simulink model "ultimate_lqr"  (R2023a)
settings: Solver=VariableStepAuto  StartTime=0.0  StopTime=10.0  RelTol=1e-3
values from neighbouring files (symbols this model uses):
  Ard = [Ar(1,1) Ar(1,3:end) ... (first row only)    [Modelo_mono.m]    (also in workspace.mat = [0 0 -31.2551437046 31.2551437046 0 0 0 0 0 0 -92.3888975157)
  Brd = [Br(1,:) ... (first row only)    [Modelo_mono.m]    (also in workspace.mat = [0  0; 0  0; 50297.8358889  0; -78.116759971  0; 0  238.3657)
  Crd = [1 0 0 0 0 0 0 1 0 0 0 0 ... (36 elements, 6x6)]    [workspace.mat]
  K = lqr(Ard,Brd,Qc,Rc)    [Modelo_mono.m]    (also in cascatinha_v3.m = [tprK,0; workspace.mat = [-891.058429104  -1.00065730536e-12  -0.217264538579  -159.5)
  v_ic = [0;0;0;0]    [Modelo_mono.m]    (also in workspace.mat = [0 0 0 0])
  x_ic = [0;5*pi/180;0;-5*pi/180]    [Modelo_mono.m]    (also in workspace.mat = [0 0.0872664625997 0 -0.0872664625997])
libraries: simulink_extras x1
settings Model: Creator=pinki  LastModifiedBy=pinki

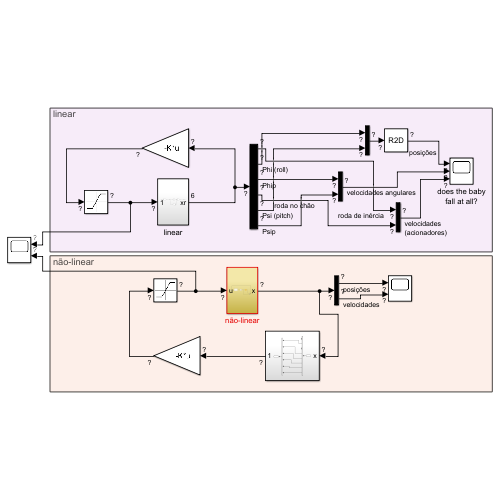
[thumbnail: Simulink's stored preview of the top-level diagram]
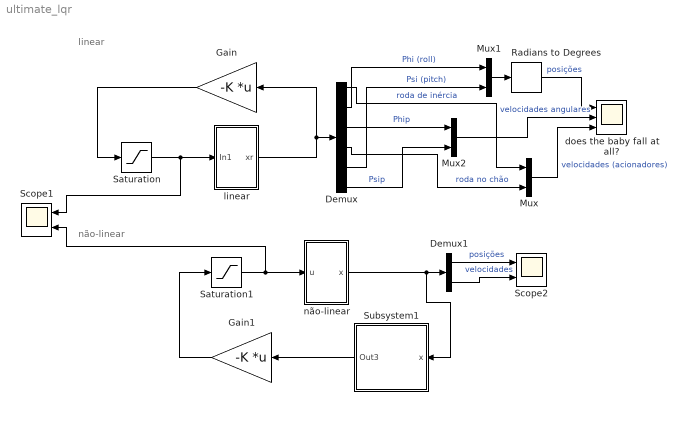
== system ultimate_lqr ==
  note: não-linear
  note: linear
  Demux : Demux  Outputs=6
  Demux1 : Demux  Outputs=2
  Gain : Gain  Gain=-K  Multiplication=Matrix(K*u)
  Gain1 : Gain  Gain=-K  Multiplication=Matrix(K*u)
  Mux : Mux  Inputs=2
  Mux1 : Mux  Inputs=2
  Mux2 : Mux  Inputs=2
  Radians to Degrees : simulink_extras/Transformations/Radians to Degrees
  Saturation : Saturate  UpperLimit=1  LowerLimit=-1
  Saturation1 : Saturate  UpperLimit=1  LowerLimit=-1
  Scope1 : Scope  NumInputPorts=2
  Scope2 : Scope  NumInputPorts=2
  Subsystem1 : Subsystem
  does the baby fall at all? : Scope  NumInputPorts=3
  linear : Subsystem
  não-linear : Subsystem
  wires:
  linear/1(xr) -> Gain/1, Demux/1
  Saturation/1 -> Scope1/1, linear/1(In1)
  Demux1/2 -> Scope2/2  "velocidades"
  Demux1/1 -> Scope2/1  "posições"
  não-linear/1(x) -> Subsystem1/1(x), Demux1/1
  Gain/1 -> Saturation/1
  Subsystem1/1(Out3) -> Gain1/1
  Gain1/1 -> Saturation1/1
  Saturation1/1 -> não-linear/1(u), Scope1/2
  Demux/1 -> Mux/1  "roda de inércia"
  Mux2/1 -> does the baby fall at all?/2  "velocidades angulares"
  Mux1/1 -> Radians to Degrees/1
  Demux/2 -> Mux1/1  "Phi (roll)"
  Mux/1 -> does the baby fall at all?/3  "velocidades (acionadores)"
  Radians to Degrees/1 -> does the baby fall at all?/1  "posições"
  Demux/4 -> Mux/2  "roda no chão"
  Demux/5 -> Mux1/2  "Psi (pitch)"
  Demux/3 -> Mux2/1  "Phip"
  Demux/6 -> Mux2/2  "Psip"

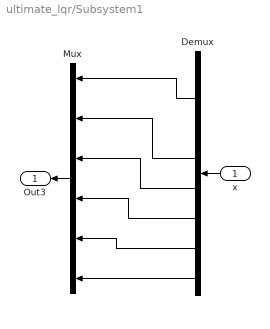
== system ultimate_lqr/Subsystem1 ==
  x : Inport
  Demux : Demux  Outputs=8
  Mux : Mux  Inputs=6
  Out3 : Outport
  wires:
  Demux/2 -> Mux/1
  Demux/4 -> Mux/2
  Demux/8 -> Mux/6
  Demux/5 -> Mux/3
  Demux/7 -> Mux/5
  Demux/6 -> Mux/4
  Mux/1 -> Out3/1
  x/1 -> Demux/1

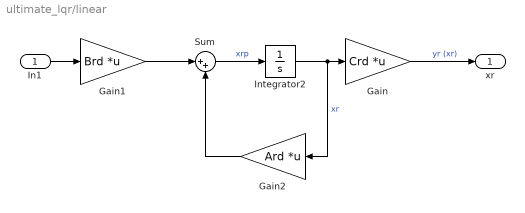
== system ultimate_lqr/linear ==
  In1 : Inport
  Gain : Gain  Gain=Crd  Multiplication=Matrix(K*u) (u vector)
  Gain1 : Gain  Gain=Brd  Multiplication=Matrix(K*u) (u vector)
  Gain2 : Gain  Gain=Ard  Multiplication=Matrix(K*u) (u vector)
  Integrator2 : Integrator  InitialCondition=x_ic
  Sum : Sum  Inputs=|++
  xr : Outport
  wires:
  Sum/1 -> Integrator2/1  "xrp"
  Gain1/1 -> Sum/1
  Gain/1 -> xr/1  "yr (xr)"
  Integrator2/1 -> Gain2/1, Gain/1  "xr"
  Gain2/1 -> Sum/2
  In1/1 -> Gain1/1

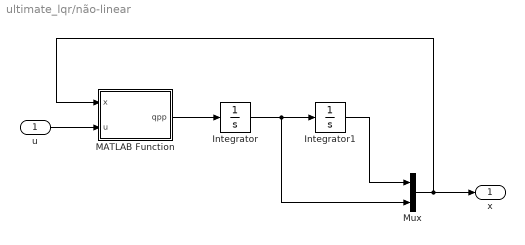
== system ultimate_lqr/não-linear ==
  u : Inport
  Integrator : Integrator  InitialCondition=v_ic
  Integrator1 : Integrator  InitialCondition=x_ic
  MATLAB Function : MATLAB Function  TreatAsAtomicUnit=on
  Mux : Mux  Inputs=2
  x : Outport
  wires:
  Integrator/1 -> Mux/2, Integrator1/1
  u/1 -> MATLAB Function/2(u)
  Mux/1 -> x/1, MATLAB Function/1(x)
  Integrator1/1 -> Mux/1
  MATLAB Function/1(qpp) -> Integrator/1

== matlab function ultimate_lqr/não-linear/MATLAB Function ==
  data: x input; u input; qpp output
function qpp = fcn(x,u)

M = function_M(x(4));
V = function_V(x(6),x(4),x(8),x(5),x(7));
G = function_G(x(2),x(4));
P = function_P();

qpp = M^-1*(-V-G+P*u);
